simulink model "obstacle_avoiding_robot"  (R2019a)
settings: Solver=FixedStepAuto  StartTime=0.0  StopTime=inf  RelTol=1e-3  EnableMultiTasking=on
libraries: arduinolib x4, LCDlib x1, arduinosensorlib x1
settings Model: ExtModeTrigDuration=2  Creator=BALAJI N V  LastModifiedBy=Dell
settings SolverCC: AutoInsertRateTranBlk=on
settings OptimizationCC: EnhancedBackFolding=on  PassReuseOutputArgsAs=Individual arguments  ZeroExternalMemoryAtStartup=off  ZeroInternalMemoryAtStartup=off  MaxStackSize=64  OptimizeBlockOrder=speed  DifferentSizesBufferReuse=on  OptimizationCustomize=off
settings DebuggingCC: ParameterTunabilityLossMsg=error
settings HardwareCC: ProdBitPerInt=16  ProdBitPerPointer=16  ProdBitPerSizeT=16  ProdBitPerPtrDiffT=16  ProdLargestAtomicFloat=None  ProdWordSize=8  ProdHWDeviceType=Atmel->AVR
settings SFSimCC: MATLABDynamicMemAlloc=off
settings RTWCC: SystemTargetFile=ert.tlc  HardwareBoard=Arduino Uno  TLCOptions=-aInlineSetEventsForThisBaseRateFcn=TLC_FALSE -aSuppressMultiTaskScheduler=TLC_FALSE -aRateBasedStepFcn=1  TemplateMakefile=ert_default_tmf  GenerateReport=on  Toolchain=Arduino AVR  BuildConfiguration=Faster Runs  IncludeHyperlinkInReport=on  LaunchReport=on  GenerateTraceInfo=on  GenerateTraceReport=on  GenerateTraceReportSl=on  GenerateTraceReportSf=on  GenerateTraceReportEml=on
settings CodeAppCC: ForceParamTrailComments=on  IgnoreCustomStorageClasses=off  OperatorAnnotations=on  SimulinkDataObjDesc=on  SFDataObjDesc=on  InsertBlockDesc=on
settings ERTTargetCC: SupportContinuousTime=on  SupportVariableSizeSignals=on  ExtModeStaticAllocSize=250

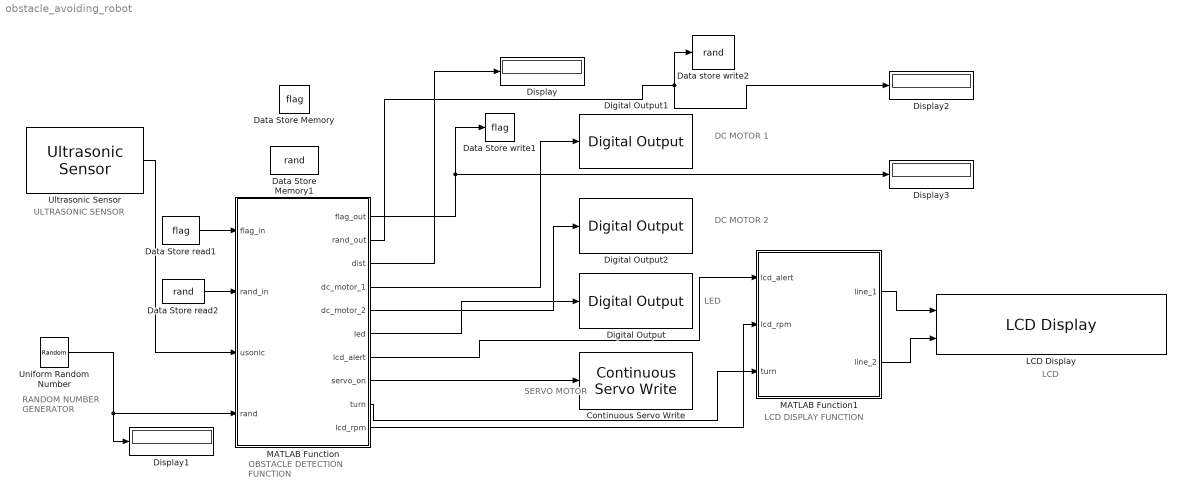
== system obstacle_avoiding_robot ==
  note: ULTRASONIC SENSOR
  note: RANDOM NUMBER
      | GENERATOR
  note: OBSTACLE DETECTION
      | FUNCTION
  note: LCD DISPLAY FUNCTION
  note: LCD
  note: LED
  note: SERVO
      | MOTOR
  note: DC MOTOR
      | 1
  note: DC MOTOR
      | 2
  Continuous Servo Write : arduinolib/Continuous Servo Write  pinNumber=10  ServoIndex=0  blockPlatform=ARDUINO
      settings: SourceProductName=Simulink Support Package for Arduino Hardware  SourceProductBaseCode=ARDUINO
  Data Store Memory : DataStoreMemory  DataStoreName=flag  ReadBeforeWriteMsg=warning  WriteAfterWriteMsg=warning  WriteAfterReadMsg=warning  ShowAdditionalParam=off
  Data Store Memory1 : DataStoreMemory  DataStoreName=rand  ReadBeforeWriteMsg=warning  WriteAfterWriteMsg=warning  WriteAfterReadMsg=warning  ShowAdditionalParam=off
  "Data Store read1 " : DataStoreRead  DataStoreName=flag
  "Data Store read2 " : DataStoreRead  DataStoreName=rand
  Data Store write1 : DataStoreWrite  DataStoreName=flag
  "Data store write2 " : DataStoreWrite  DataStoreName=rand
  Digital Output : arduinolib/Digital Output  pinNumber=13  blockPlatform=arduino
  Digital Output1 : arduinolib/Digital Output  pinNumber=6  blockPlatform=arduino
  Digital Output2 : arduinolib/Digital Output  pinNumber=7  blockPlatform=arduino
  Display{,1..3} (4 alike) : Display
  LCD Display : LCDlib/LCD Display  pins=[12,11,5, 4, 3, 2]
      settings: SourceProductName=LCD Library
  MATLAB Function : MATLAB Function  TreatAsAtomicUnit=on
  MATLAB Function1 : MATLAB Function  TreatAsAtomicUnit=on
  Ultrasonic Sensor : arduinosensorlib/Ultrasonic Sensor  NumSignalPins=2  TrigPin=8  EchoPin=9  SignalPin=9  SampleTime_=0.3  blockPlatform=ARDUINO
      settings: SourceProductName=Simulink Support Package for Arduino Hardware  SourceProductBaseCode=ARDUINO
  Uniform Random Number : UniformRandomNumber  SampleTime=0.3
  wires:
  Ultrasonic Sensor/1 -> MATLAB Function/3(usonic)
  MATLAB Function/3(dist) -> Display/1
  Uniform Random Number/1 -> Display1/1, MATLAB Function/4(rand)
  MATLAB Function/6(led) -> Digital Output/1
  MATLAB Function/5(dc_motor_2) -> Digital Output2/1
  MATLAB Function1/1(line_1) -> LCD Display/1
  MATLAB Function1/2(line_2) -> LCD Display/2
  MATLAB Function/7(lcd_alert) -> MATLAB Function1/1(lcd_alert)
  MATLAB Function/9(turn) -> MATLAB Function1/3(turn)
  MATLAB Function/10(lcd_rpm) -> MATLAB Function1/2(lcd_rpm)
  "Data Store read1 "/1 -> MATLAB Function/1(flag_in)
  "Data Store read2 "/1 -> MATLAB Function/2(rand_in)
  MATLAB Function/1(flag_out) -> Data Store write1/1, Display3/1
  MATLAB Function/2(rand_out) -> Display2/1, "Data store write2 "/1
  MATLAB Function/4(dc_motor_1) -> Digital Output1/1
  MATLAB Function/8(servo_on) -> Continuous Servo Write/1

== matlab function obstacle_avoiding_robot/MATLAB Function1 ==
  data: lcd_alert input; line_1 output; lcd_rpm input; turn input; line_2 output
function [line_1,line_2] = lcd_fn(lcd_alert,lcd_rpm,turn)
if(lcd_rpm==1 && lcd_alert==0) % Cases where obstacle detected or not.
    while 1
    line_1=[[82],[80],[77],[33],[33]]; % "RPM!!" in ASCII 
    pause(0.5);
    line_1=[[32]]
else
    line_1=[[65],[76],[69],[82],[84]]; % "ALERT" in ASCII
end
    switch turn % switch case works for clockwise,anticlockwise motions of the servo arm and also to display the rpm value of the dc motor 
        case 0
        line_2=[[84],[85],[82],[78],[73],[78],[71],[33],[76],[69],[70],[84],[33]]; % "TURNING LEFT" in ASCII
        case 1
        line_2=[[84],[85],[82],[78],[73],[78],[71],[33],[82],[73],[71],[72],[84]]; % "TURNING RIGHT" in ASCII
        case 2
        line_2=[[51],[48],[48],[32],[32],[32],[32],[32],[32],[32],[32],[32],[32]]; % "300" rpm value in ASCII
        otherwise
          line_2=[[51],[48],[48],[32],[32],[32],[32],[32],[32],[32],[32],[32],[32]]; % "300" rpm value in ASCII 
    end
end

== matlab function obstacle_avoiding_robot/MATLAB Function ==
  data: flag_in input; rand_in input; flag_out output; rand_out output; usonic input; dist output; rand input; dc_motor_1 output; dc_motor_2 output; led output; lcd_alert output; servo_on output; turn output; lcd_rpm output
function [flag_out,rand_out,dist,dc_motor_1,dc_motor_2,led,lcd_alert,servo_on,turn,lcd_rpm]  = od(flag_in,rand_in,usonic,rand)
dist=usonic/0.0686;% Conversion to distance(cm)
if(dist>0 && dist<=3)
    lcd_alert=1; % 'ALERT' to enable its functionality in lcd_fn
    lcd_rpm=0; % 'rpm' to enable its functionality in lcd_fn
    led=1; 
    dc_motor_1=0; % output 1 of dc motor which later goes to DC motor driver to run/stop the motor
    dc_motor_2=0; % output 2 of dc motor dc motor which later goes to DC motor driver to run/stop the motor
    turn=2; % switches to Case 2 in the 'lcd_fn'
    if(flag_in==0) % initial condition check
        rand_out=rand; % rand value to the data write block
        flag_out=1; % flag is 1 when there is an obstacle
        if(rand_out>0) % checking rand value
        servo_on=[90]; % rotates servo to 90 degrees
        turn=1; % right turn
        else
            servo_on=[-90]; % rotates to -90 degrees
            turn=0; % left turn
        end
    else 
        if(rand_in>0)
        servo_on=[90];  % rotates servo to 90 degrees
        turn=1; % right turn
        else
            servo_on=[-90]; %  rotates to -90 degrees
            turn=0; % left turn
        end
        flag_out=1; % flag=1 and else condition starts working
        rand_out=rand_in; % stored rand number remains unchanged until the obstacle is removed
    end
 else
    servo_on=[30];
    pause(2)
    servo_on=[-90];
    flag_out=0; % flag=0 implies that intial value stored to the flag
    rand_out=rand; % rand_out is updated
    lcd_alert=0;
    led=0;
    dc_motor_1=1; % output 1 of dc motor 
    dc_motor_2=0; % output 2 of dc motor
    lcd_rpm=1;
    turn=2;
end
